simulink model "dsss"  (Simulink 7.1)
settings: Solver=ode45  StartTime=0.0  StopTime=0.80  RelTol=1e-3
libraries: simulink x264, dspbuff3 x24, dspxfrm3 x8, commsynccomp2 x5, dspsigops x4, dspobslib x4, dsparch4 x3, commutil2 x2, commseqgen2 x1, commfilt2 x1, commsink2 x1, dspspect3 x1
(part 1 of 4)
settings Model: Creator=Administrator  LastModifiedBy=Administrator

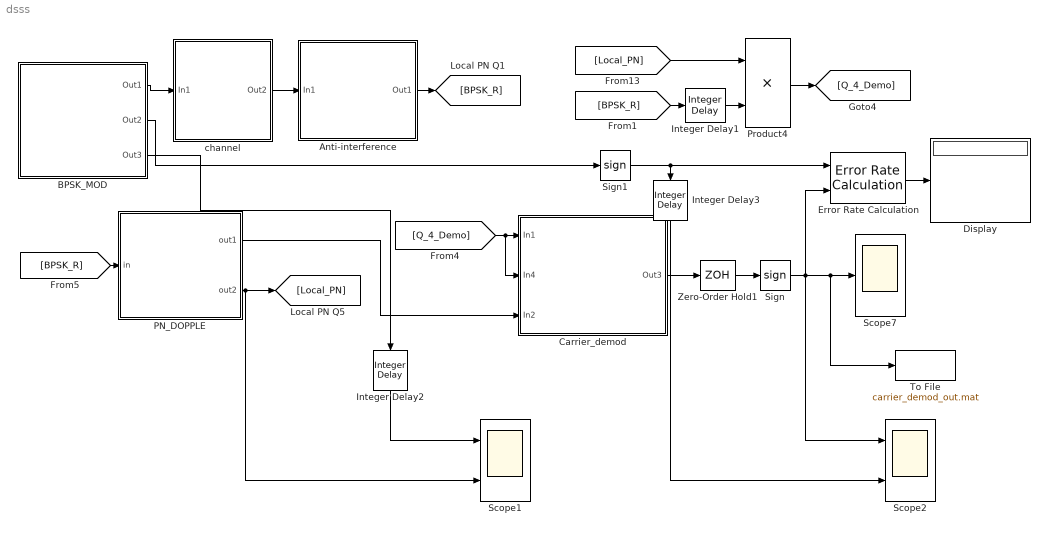
== system dsss ==
  Anti-interference : Subsystem
  BPSK_MOD : Subsystem
  Carrier_demod : Subsystem
  Display : Display
  Error Rate Calculation : commsink2/Error Rate Calculation  N=5  st_delay=0  cp_mode=Entire frame  subframe=[]  PMode=Port  WsName=ErrorVec  RsMode2=off  stop=off  numErr=100  maxBits=1e6
  Integer Delay1 : simulink/Discrete/Integer Delay  vinit=0.0  samptime=1/5.1e6  NumDelays=172
  Integer Delay2 : simulink/Discrete/Integer Delay  Orientation=down  vinit=0.0  samptime=1/5.1e6  NumDelays=22700
  Integer Delay3 : simulink/Discrete/Integer Delay  Orientation=down  vinit=0.0  samptime=1/1000  NumDelays=5
  PN_DOPPLE : Subsystem  TreatAsAtomicUnit=on
  Product4 : Product  OutDataType=sfix(16)  OutScaling=2^0  RndMeth=Zero
  Scope1 : Scope  NumInputPorts=2
      settings: YMin=-5~-5  YMax=5~5  SaveName=ScopeData3  MaxDataPoints=100000
  Scope2 : Scope  NumInputPorts=2
      settings: YMin=-5~-5  YMax=5~5  SaveName=ScopeData5  MaxDataPoints=100000
  Scope7 : Scope
      settings: SaveName=ScopeData7  MaxDataPoints=100000
  Sign : Signum
  Sign1 : Signum
  To File : ToFile  Filename=carrier_demod_out.mat
  Zero-Order Hold1 : ZeroOrderHold  SampleTime=1/1e3
  channel : Subsystem
  wires:
  BPSK_MOD/1(Out1) -> channel/1(In1)
  [BPSK_R] -> PN_DOPPLE/1(in)
  [Local_PN] -> Product4/1
  Product4/1 -> [Q_4_Demo]
  [BPSK_R] -> Integer Delay1/1
  Integer Delay1/1 -> Product4/2
  [Q_4_Demo] -> Carrier_demod/2(In4), Carrier_demod/1(In1)
  Carrier_demod/1(Out3) -> Zero-Order Hold1/1
  Zero-Order Hold1/1 -> Sign/1
  PN_DOPPLE/1(out1) -> Carrier_demod/3(In2)
  Sign/1 -> Error Rate Calculation/2, Scope2/1, Scope7/1, To File/1
  channel/1(Out2) -> Anti-interference/1(In1)
  Anti-interference/1(Out1) -> [BPSK_R]
  Error Rate Calculation/1 -> Display/1
  BPSK_MOD/2(Out2) -> Sign1/1
  PN_DOPPLE/2(out2) -> [Local_PN], Scope1/2
  BPSK_MOD/3(Out3) -> Integer Delay2/1
  Integer Delay2/1 -> Scope1/1
  Integer Delay3/1 -> Scope2/2
  Sign1/1 -> Error Rate Calculation/1, Integer Delay3/1

== system dsss/Anti-interference ==
  In1 : Inport  OutDataType=sfix(16)  OutScaling=2^0
  Add1 : Sum  Inputs=++++  OutDataType=sfix(16)  OutScaling=2^-10
  firstroad : Subsystem
  firstroad1 : Subsystem
  firstroad2 : Subsystem
  firstroad3 : Subsystem
  Out1 : Outport  OutDataType=sfix(16)  OutScaling=2^0
  wires:
  firstroad/1(Out1) -> Add1/1
  firstroad1/1(Out1) -> Add1/2
  firstroad2/1(Out1) -> Add1/3
  firstroad3/1(Out1) -> Add1/4
  In1/1 -> firstroad/1(In1), firstroad1/1(In1), firstroad2/1(In1), firstroad3/1(In1)
  Add1/1 -> Out1/1

== system dsss/BPSK_MOD ==
  Continuous-Time VCO1 : commsynccomp2/Continuous-Time VCO  SystemSampleTime=-1  Ac=1  Fc=510000  Kc=1000  Ph=pi/2
  PN_MOD : Subsystem
  Product6 : Product  OutDataType=sfix(16)  OutScaling=2^0  RndMeth=Zero
  Zero-Order Hold3 : ZeroOrderHold  SampleTime=1/5.1e6
  Out1 : Outport  OutDataType=sfix(16)  OutScaling=2^0
  Out2 : Outport  Port=2  OutDataType=sfix(16)  OutScaling=2^0
  Out3 : Outport  Port=3  OutDataType=sfix(16)  OutScaling=2^0
  wires:
  PN_MOD/1(Out1) -> Product6/2
  Continuous-Time VCO1/1 -> Zero-Order Hold3/1
  Zero-Order Hold3/1 -> Product6/1
  Product6/1 -> Out1/1
  PN_MOD/2(Out2) -> Out2/1
  PN_MOD/3(Out3) -> Out3/1

== system dsss/Carrier_demod ==
  note: 1.27e6 Hz
      |
      | 1/10.2e6
      |
      | 255K-300K
  In1 : Inport  OutDataType=sfix(16)  OutScaling=2^0
  In4 : Inport  Port=2  OutDataType=sfix(16)  OutScaling=2^0
  In2 : Inport  Port=3  OutDataType=sfix(16)  OutScaling=2^0
  Abs : Abs
  Add2 : Sum  Orientation=left  OutDataType=sfix(16)  OutScaling=2^-10
  Constant2 : Constant  OutDataType=sfix(16)  OutScaling=2^0
  Continuous-Time CO1 : commsynccomp2/Continuous-Time VCO  Orientation=left  SystemSampleTime=-1  Ac=2  Fc=5.1e5  Kc=1000  Ph=0
  Continuous-Time CO2 : commsynccomp2/Continuous-Time VCO  Orientation=left  SystemSampleTime=-1  Ac=2  Fc=5.1e5  Kc=1000  Ph=pi/2
  Digital Filter Design1 : dsparch4/Digital Filter Design  SystemSampleTime=-1  mwdsp_browser_bugfix_var=off
  Digital Filter Design2 : dsparch4/Digital Filter Design  SystemSampleTime=-1  mwdsp_browser_bugfix_var=off
  LF : Subsystem  Orientation=left
  Product : Product  OutDataType=sfix(16)  OutScaling=2^0  SaturateOnIntegerOverflow=on  OutDataTypeStr=Inherit: Same as first input
  Product2 : Product  Orientation=left  OutDataType=sfix(16)  OutScaling=2^0  SaturateOnIntegerOverflow=on  OutDataTypeStr=Inherit: Same as first input
  Product4 : Product  OutDataType=sfix(16)  OutScaling=2^0  SaturateOnIntegerOverflow=on  OutDataTypeStr=Inherit: Same as first input
  Scope{1..5} (5 alike) : Scope
      Scope1 settings: TimeRange=0.06427185951473757  YMin=-2  YMax=2  MaxDataPoints=100000
      Scope2 settings: TimeRange=0.06427185951473757  YMin=-2  YMax=2  SaveName=ScopeData6  MaxDataPoints=100000
      Scope3 settings: YMin=-2  YMax=2  SaveName=ScopeData35
      Scope4 settings: TimeRange=0.06427185951473757  YMin=-2  YMax=2  SaveName=ScopeData8  MaxDataPoints=100000
      Scope5 settings: TimeRange=0.06427185951473757  YMin=-2  YMax=2  SaveName=ScopeData2  MaxDataPoints=100000
  Subsystem2 : Subsystem  TreatAsAtomicUnit=on
  Switch2 : Switch  Criteria=u2 > Threshold
  Zero-Order Hold3 : ZeroOrderHold  Orientation=up  SampleTime=1/5.1e6
  Zero-Order Hold4 : ZeroOrderHold  SampleTime=1/1e5
  Zero-Order Hold5 : ZeroOrderHold  Orientation=down  SampleTime=1/5.1e6
  Zero-Order Hold6 : ZeroOrderHold  SampleTime=1/5.1e6
  Out3 : Outport  OutDataType=sfix(16)  OutScaling=2^0
  wires:
  Product2/1 -> LF/1(In2)
  Product/1 -> Digital Filter Design2/1
  Continuous-Time CO1/1 -> Zero-Order Hold3/1
  Digital Filter Design2/1 -> Product2/1, Abs/1, Zero-Order Hold6/1, Scope1/1  "unmoduled signal"
  In1/1 -> Product/1
  LF/1(Out1) -> Scope2/1, Add2/1
  Zero-Order Hold3/1 -> Product/2
  Subsystem2/1(Out1) -> Out3/1
  Constant2/1 -> Switch2/1
  Zero-Order Hold4/1 -> Switch2/2
  Switch2/1 -> Scope3/1, Subsystem2/Enable
  Abs/1 -> Zero-Order Hold4/1
  Zero-Order Hold6/1 -> Subsystem2/1(In1)
  Digital Filter Design1/1 -> Product2/2, Scope5/1
  Continuous-Time CO2/1 -> Zero-Order Hold5/1
  Product4/1 -> Digital Filter Design1/1
  In4/1 -> Product4/2
  Zero-Order Hold5/1 -> Product4/1
  Add2/1 -> Continuous-Time CO1/1, Continuous-Time CO2/1
  In2/1 -> Scope4/1, Add2/2

== system dsss/PN_DOPPLE ==
  in : Inport  OutDataType=sfix(16)  OutScaling=2^0
  "De-Carrier " : Subsystem
  FFT compensate : Subsystem
  Local PN : Subsystem
  MF Subsystem : Subsystem
  Magnitude FFT2 : dspspect3/Magnitude FFT  SystemSampleTime=-1  mag_or_magsq=Magnitude  fftLenInherit=off  fftsize=32
  MainTain System : Subsystem  TreatAsAtomicUnit=on
  Scope1 : Scope
      settings: TimeRange=0.06427185951473757  YMin=-2  YMax=2  SaveName=ScopeData14  MaxDataPoints=100000
  Scope3 : Scope
      settings: TimeRange=0.06427185951473757  YMin=-2  YMax=2  SaveName=ScopeData45  MaxDataPoints=100000
  Scope4 : Scope
      settings: TimeRange=0.06427185951473757  YMin=-2  YMax=2  SaveName=ScopeData21  MaxDataPoints=100000
  Sign : Signum
  Zero-Order Hold : ZeroOrderHold  SampleTime=1/255e3
  out1 : Outport  OutDataType=sfix(16)  OutScaling=2^0
  out2 : Outport  Port=2  OutDataType=sfix(16)  OutScaling=2^0
  wires:
  in/1 -> "De-Carrier "/1(in)
  FFT compensate/2(PN Peak) -> Scope3/1, Local PN/1(in)
  Zero-Order Hold/1 -> Sign/1, Scope4/1
  Sign/1 -> MF Subsystem/1(In1), Scope1/1, Local PN/2(in1)
  MF Subsystem/1(bus Out1) -> Magnitude FFT2/1
  Magnitude FFT2/1 -> FFT compensate/1(In1)
  FFT compensate/1(FFT compensate positive) -> MainTain System/1(In1), MainTain System/Trigger
  MainTain System/1(Out1) -> out1/1
  "De-Carrier "/1(out) -> Zero-Order Hold/1
  Local PN/1(1 0 0 1 1 1 0 1) -> out2/1

== system dsss/channel ==
  In1 : Inport  OutDataType=sfix(16)  OutScaling=2^0
  AWGN Channel : commchan3/AWGN Channel  SystemSampleTime=-1  seed=67  noiseMode="Signal to noise ratio  (SNR)"  EbNodB=10  EsNodB=10  SNRdB=-3.95  bitsPerSym=1  Ps=1  Tsym=1  variance=1
  Add : Sum  OutDataType=sfix(16)  OutScaling=2^-10
  Scope9 : Scope
      settings: TimeRange=0.06427185951473757  YMin=0  YMax=14
  Zero-Order Hold1 : ZeroOrderHold  SampleTime=1/5.1e6
  Zero-Order Hold3 : ZeroOrderHold  SampleTime=1/5.1e6
  zhaidaigr : Subsystem
  Out2 : Outport  OutDataType=sfix(16)  OutScaling=2^0
  wires:
  Zero-Order Hold3/1 -> Scope9/1, AWGN Channel/1
  In1/1 -> Zero-Order Hold3/1
  zhaidaigr/1(Out1) -> Add/2
  Add/1 -> Out2/1
  Zero-Order Hold1/1 -> Add/1
  AWGN Channel/1 -> Zero-Order Hold1/1

== system dsss/Anti-interference/firstroad ==
  In1 : Inport  OutDataType=sfix(16)  OutScaling=2^0
  Complex to Magnitude-Angle : ComplexToMagnitudeAngle
  all : Subsystem
  inteference_delieve : Subsystem
  inverse_convertion : Subsystem  Orientation=left
  threshold : Subsystem
  Out1 : Outport  Orientation=left  OutDataType=sfix(16)  OutScaling=2^0
  wires:
  all/1(Out1) -> Complex to Magnitude-Angle/1
  Complex to Magnitude-Angle/1 -> threshold/1(In1), inteference_delieve/1(In1)
  Complex to Magnitude-Angle/2 -> inverse_convertion/1(In1)
  inteference_delieve/1(Out1) -> inverse_convertion/2(In2)
  threshold/1(Out1) -> inteference_delieve/2(In2)
  In1/1 -> all/1(In1)
  inverse_convertion/1(Out1) -> Out1/1

== system dsss/Anti-interference/firstroad1 ==
  In1 : Inport  OutDataType=sfix(16)  OutScaling=2^0
  Complex to Magnitude-Angle : ComplexToMagnitudeAngle
  all : Subsystem
  inteference_delieve : Subsystem
  inverse_convertion : Subsystem  Orientation=left
  threshold : Subsystem
  Out1 : Outport  Orientation=left  OutDataType=sfix(16)  OutScaling=2^0
  wires:
  inverse_convertion/1(Out1) -> Out1/1
  In1/1 -> all/1(In1)
  threshold/1(Out1) -> inteference_delieve/2(In2)
  inteference_delieve/1(Out1) -> inverse_convertion/2(In2)
  Complex to Magnitude-Angle/2 -> inverse_convertion/1(In1)
  Complex to Magnitude-Angle/1 -> inteference_delieve/1(In1), threshold/1(In1)
  all/1(Out1) -> Complex to Magnitude-Angle/1

== system dsss/Anti-interference/firstroad2 ==
  In1 : Inport  OutDataType=sfix(16)  OutScaling=2^0
  Complex to Magnitude-Angle : ComplexToMagnitudeAngle
  all : Subsystem
  inteference_delieve : Subsystem
  inverse_convertion : Subsystem  Orientation=left
  threshold : Subsystem
  Out1 : Outport  Orientation=left  OutDataType=sfix(16)  OutScaling=2^0
  wires:
  all/1(Out1) -> Complex to Magnitude-Angle/1
  Complex to Magnitude-Angle/1 -> threshold/1(In1), inteference_delieve/1(In1)
  Complex to Magnitude-Angle/2 -> inverse_convertion/1(In1)
  inteference_delieve/1(Out1) -> inverse_convertion/2(In2)
  threshold/1(Out1) -> inteference_delieve/2(In2)
  In1/1 -> all/1(In1)
  inverse_convertion/1(Out1) -> Out1/1

== system dsss/Anti-interference/firstroad3 ==
  In1 : Inport  OutDataType=sfix(16)  OutScaling=2^0
  Complex to Magnitude-Angle : ComplexToMagnitudeAngle
  all : Subsystem
  inteference_delieve : Subsystem
  inverse_convertion : Subsystem  Orientation=left
  threshold : Subsystem
  Out1 : Outport  Orientation=left  OutDataType=sfix(16)  OutScaling=2^0
  wires:
  inverse_convertion/1(Out1) -> Out1/1
  In1/1 -> all/1(In1)
  threshold/1(Out1) -> inteference_delieve/2(In2)
  inteference_delieve/1(Out1) -> inverse_convertion/2(In2)
  Complex to Magnitude-Angle/2 -> inverse_convertion/1(In1)
  Complex to Magnitude-Angle/1 -> inteference_delieve/1(In1), threshold/1(In1)
  all/1(Out1) -> Complex to Magnitude-Angle/1

== system dsss/BPSK_MOD/PN_MOD ==
  1 0 0 0 1 1 1 0 2 : commseqgen2/PN Sequence Generator  poly=[1 0 0 0 1 1 1 0 1]  ini_sta=[0 0 0 0 0 0 0 1]  outBitMaskSource=Dialog parameter  shift=0  Ts=1/2.55e5  frameBased=off  sampPerFrame=1  reset=off  bitPackedOutputs=off  outDataType=double  numPackedBits=8  bitPackDataSigned=off  bitPackedOutDType=double
  From File : FromFile  FileName=encode_out.mat  SampleTime=1/1000
  Product5 : Product  OutDataType=sfix(16)  OutScaling=2^0  RndMeth=Zero
  Unipolar to Bipolar Converter : commutil2/Unipolar to Bipolar Converter  SystemSampleTime=-1  M=2  polarity=Positive  dataType=Same as input
  Out1 : Outport
  Out2 : Outport  Port=2
  Out3 : Outport  Port=3
  wires:
  1 0 0 0 1 1 1 0 2/1 -> Unipolar to Bipolar Converter/1
  Unipolar to Bipolar Converter/1 -> Product5/1, Out3/1
  From File/1 -> Product5/2, Out2/1
  Product5/1 -> Out1/1

== system dsss/Carrier_demod/LF ==
  In2 : Inport  OutDataType=sfix(16)  OutScaling=2^0
  Gain : Gain  Gain=0.4  ParameterDataType=sfix(16)  ParameterScaling=2^0  OutDataType=sfix(16)  OutScaling=2^0  SaturateOnIntegerOverflow=on  OutDataTypeStr=Inherit: Same as input  ParamDataTypeStr=Inherit: Same as input
  Gain1 : Gain  Gain=0.02  ParameterDataType=sfix(16)  ParameterScaling=2^0  OutDataType=sfix(16)  OutScaling=2^0  SaturateOnIntegerOverflow=on  OutDataTypeStr=Inherit: Same as input  ParamDataTypeStr=Inherit: Same as input
  Sum1 : Sum  Inputs=|++  OutDataType=sfix(16)  OutScaling=2^0  SaturateOnIntegerOverflow=on  InputSameDT=on  OutDataTypeStr=Inherit: Same as first input
  Sum2 : Sum  Inputs=|++  OutDataType=sfix(16)  OutScaling=2^0  SaturateOnIntegerOverflow=on  InputSameDT=on  OutDataTypeStr=Inherit: Same as first input
  Unit Delay : UnitDelay  Orientation=left  SampleTime=1/1e5
  Out1 : Outport  OutDataType=sfix(16)  OutScaling=2^0
  wires:
  In2/1 -> Gain1/1, Gain/1
  Gain1/1 -> Sum2/1
  Unit Delay/1 -> Sum2/2
  Gain/1 -> Sum1/1
  Sum1/1 -> Out1/1
  Sum2/1 -> Sum1/2, Unit Delay/1

== system dsss/Carrier_demod/Subsystem2 ==
  In1 : Inport  OutDataType=sfix(16)  OutScaling=2^0
  Enable : EnablePort
  Gain : Gain  Gain=1/100  ParameterDataType=sfix(16)  ParameterScaling=2^0  OutDataType=sfix(16)  OutScaling=2^0
  Integrate and Dump : commfilt2/Integrate and Dump  DialogController=commDDGCreate  DialogControllerArgs=DataTag18  obssamples=100  offsetsamples=0  nodump=off  roundingMode=Floor  overflowMode=off
  Out1 : Outport  OutDataType=sfix(16)  OutScaling=2^0
  wires:
  Integrate and Dump/1 -> Gain/1
  In1/1 -> Integrate and Dump/1
  Gain/1 -> Out1/1

== system dsss/PN_DOPPLE/De-Carrier  ==
  note: 5.1e5 Hz
      |
      | 1/5.1e6
      |
      | 255K-300K
  in : Inport  OutDataType=sfix(16)  OutScaling=2^0
  Continuous-Time VCO1 : commsynccomp2/Continuous-Time VCO  SystemSampleTime=-1  Ac=1  Fc=5.1e5  Kc=1000  Ph=pi/2
  Digital Filter Design4 : dsparch4/Digital Filter Design  SystemSampleTime=-1  mwdsp_browser_bugfix_var=off
  Product1 : Product  OutDataType=sfix(16)  OutScaling=2^0  RndMeth=Zero
  Scope1 : Scope
      settings: SaveName=ScopeData4  MaxDataPoints=100000
  Scope3 : Scope
      settings: SaveName=ScopeData16  MaxDataPoints=100000
  Zero-Order Hold2 : ZeroOrderHold  SampleTime=1/5.1e6
  out : Outport  OutDataType=sfix(16)  OutScaling=2^0
  wires:
  in/1 -> Product1/2
  Product1/1 -> Scope3/1, Digital Filter Design4/1
  Digital Filter Design4/1 -> out/1, Scope1/1
  Continuous-Time VCO1/1 -> Zero-Order Hold2/1
  Zero-Order Hold2/1 -> Product1/1

== system dsss/PN_DOPPLE/FFT compensate ==
  In1 : Inport  OutDataType=sfix(16)  OutScaling=2^0
  Demux : Demux  Outputs=32
  Product1 : Product  OutDataType=sfix(16)  OutScaling=2^0  RndMeth=Zero
  Product8 : Product  OutDataType=sfix(16)  OutScaling=2^0  RndMeth=Zero
  Rate Transition1 : RateTransition  Deterministic=off  OutPortSampleTime=1/5.1e6
  Rate Transition2 : RateTransition  Deterministic=off  OutPortSampleTime=1/5.1e6
  Rate Transition3 : RateTransition  Deterministic=off  OutPortSampleTime=1/5.1e6
  Scope{1..2,4..7} (6 alike) : Scope  NumInputPorts=3
      Scope1 settings: TimeRange=0.06427185951473757  YMin=0~-5~-5  YMax=14~5~5  SaveName=ScopeData9  MaxDataPoints=100000
      Scope2 settings: TimeRange=0.06427185951473757  YMin=0~-5~-5  YMax=14~5~5  SaveName=ScopeData11  MaxDataPoints=100000
      Scope4 settings: TimeRange=0.06427185951473757  YMin=0~-5~-5  YMax=14~5~5  SaveName=ScopeData12  MaxDataPoints=100000
      Scope5 settings: TimeRange=0.06427185951473757  YMin=0~-5~-5  YMax=14~5~5  SaveName=ScopeData13  MaxDataPoints=100000
      Scope6 settings: TimeRange=0.06427185951473757  YMin=0~-5~-5  YMax=14~5~5  SaveName=ScopeData33  MaxDataPoints=100000
      Scope7 settings: TimeRange=0.06427185951473757  YMin=0~-5~-5  YMax=14~5~5  SaveName=ScopeData47  MaxDataPoints=100000
  Scope14 : Scope
      settings: SaveName=ScopeData24  MaxDataPoints=100000
  Scope3 : Scope
      settings: SaveName=ScopeData27  MaxDataPoints=100000
  Step : Step  Time=0.001  SampleTime=0
  Step1 : Step  Time=0.001  SampleTime=0
  Subsystem : Subsystem
  FFT compensate positive : Outport  OutDataType=sfix(16)  OutScaling=2^0
  PN Peak : Outport  Port=2  OutDataType=sfix(16)  OutScaling=2^0
  wires:
  Demux/3 -> Subsystem/3(In3), Scope2/3
  Demux/2 -> Subsystem/2(In2), Scope2/2
  Demux/4 -> Scope1/1, Subsystem/4(In4)
  Demux/5 -> Scope1/2, Subsystem/5(In5)
  Demux/6 -> Scope1/3, Subsystem/6(In6)
  Demux/7 -> Subsystem/7(In7), Scope4/1
  Demux/8 -> Subsystem/8(In8), Scope4/2
  Demux/9 -> Subsystem/9(In9), Scope4/3
  Demux/10 -> Subsystem/10(In10), Scope5/1
  Demux/11 -> Subsystem/11(In11), Scope5/2
  Demux/12 -> Subsystem/12(In12), Scope5/3
  Demux/13 -> Subsystem/13(In13), Scope6/1
  Demux/14 -> Subsystem/14(In14), Scope6/2
  Demux/15 -> Subsystem/15(In15), Scope6/3
  In1/1 -> Demux/1
  Demux/1 -> Subsystem/1(In1), Scope2/1
  Subsystem/1(Out1) -> Scope14/1, Product1/1
  Step/1 -> Rate Transition3/1
  Product8/1 -> Rate Transition1/1
  Subsystem/2(Out2) -> Rate Transition2/1
  Rate Transition1/1 -> PN Peak/1, Scope3/1
  Rate Transition2/1 -> Product8/1
  Demux/16 -> Subsystem/16(In16), Scope7/1
  Demux/17 -> Scope7/2
  Demux/18 -> Scope7/3
  Rate Transition3/1 -> Product8/2
  Step1/1 -> Product1/2
  Product1/1 -> FFT compensate positive/1

== system dsss/PN_DOPPLE/Local PN ==
  in : Inport  OutDataType=sfix(16)  OutScaling=2^0
  in1 : Inport  Port=2  OutDataType=sfix(16)  OutScaling=2^0
  Scope{1..3,5} (4 alike) : Scope
      Scope1 settings: TimeRange=0.06427185951473757  YMin=-2  YMax=2  SaveName=ScopeData23  MaxDataPoints=100000
      Scope2 settings: TimeRange=0.06427185951473757  YMin=-2  YMax=2  SaveName=ScopeData29  MaxDataPoints=100000
      Scope3 settings: TimeRange=0.06427185951473757  YMin=-2  YMax=2  SaveName=ScopeData18  MaxDataPoints=100000
      Scope5 settings: TimeRange=0.06427185951473757  YMin=-2  YMax=2  SaveName=ScopeData30  MaxDataPoints=100000
  local PN sequence Include Track : Subsystem  TreatAsAtomicUnit=on
  logic control : Subsystem  TreatAsAtomicUnit=on
  threshold deside : Subsystem  TreatAsAtomicUnit=on
  threshold deside stop and start : Subsystem
  1 0 0 1 1 1 0 1 : Outport  OutDataType=sfix(16)  OutScaling=2^0
  wires:
  logic control/1(Out2) -> Scope5/1, local PN sequence Include Track/Enable
  threshold deside/1(Out2) -> logic control/1(In1), threshold deside stop and start/1(In1)
  threshold deside stop and start/1(Out1) -> threshold deside/Enable, Scope3/1
  [A] -> threshold deside stop and start/2(In2)
  in/1 -> threshold deside/1(In1), Scope2/1
  local PN sequence Include Track/1("1 0 0 1 1 1 0 1 ") -> 1 0 0 1 1 1 0 1/1, Scope1/1
  ? -> local PN sequence Include Track/1(B)

== system dsss/PN_DOPPLE/MF Subsystem ==
  In1 : Inport  OutDataType=sfix(16)  OutScaling=2^0
  Add : Sum  Inputs=++++++++++++++++++++++++++++++++  OutDataType=sfix(16)  OutScaling=2^-10
  MF array : Subsystem
  Mux : Mux  Inputs=32
  Scope14 : Scope
      settings: SaveName=ScopeData34  MaxDataPoints=100000
  Zero-Order Hold : ZeroOrderHold  SampleTime=1/255000
  bus Out1 : Outport  OutDataType=sfix(16)  OutScaling=2^0
  wires:
  In1/1 -> Zero-Order Hold/1
  Zero-Order Hold/1 -> MF array/1(In1)
  Mux/1 -> bus Out1/1
  Add/1 -> Scope14/1
  MF array/1(Out1) -> Mux/1, Add/1
  MF array/2(Out2) -> Mux/2, Add/2
  MF array/3(Out3) -> Mux/3, Add/3
  MF array/4(Out4) -> Mux/4, Add/4
  MF array/5(Out5) -> Mux/5, Add/5
  MF array/6(Out6) -> Mux/6, Add/6
  MF array/7(Out7) -> Mux/7, Add/7
  MF array/8(Out8) -> Mux/8, Add/8
  MF array/9(Out9) -> Mux/9, Add/9
  MF array/10(Out10) -> Mux/10, Add/10
  MF array/11(Out11) -> Mux/11, Add/11
  MF array/12(Out12) -> Mux/12, Add/12
  MF array/13(Out13) -> Mux/13, Add/13
  MF array/14(Out14) -> Mux/14, Add/14
  MF array/15(Out15) -> Mux/15, Add/15
  MF array/16(Out16) -> Mux/16, Add/16
  MF array/17(Out17) -> Mux/17, Add/17
  MF array/18(Out18) -> Mux/18, Add/18
  MF array/19(Out19) -> Mux/19, Add/19
  MF array/20(Out20) -> Mux/20, Add/20
  MF array/21(Out21) -> Mux/21, Add/21
  MF array/22(Out22) -> Mux/22, Add/22
  MF array/23(Out23) -> Mux/23, Add/23
  MF array/24(Out24) -> Mux/24, Add/24
  MF array/25(Out25) -> Mux/25, Add/25
  MF array/26(Out26) -> Mux/26, Add/26
  MF array/27(Out27) -> Mux/27, Add/27
  MF array/28(Out28) -> Mux/28, Add/28
  MF array/29(Out29) -> Mux/29, Add/29
  MF array/30(Out30) -> Mux/30, Add/30
  MF array/31(Out31) -> Mux/31, Add/31
  MF array/32(Out32) -> Mux/32, Add/32

== system dsss/PN_DOPPLE/MainTain System ==
  In1 : Inport  OutDataType=sfix(16)  OutScaling=2^0
  Trigger : TriggerPort
  Out1 : Outport  OutDataType=sfix(16)  OutScaling=2^0
  wires:
  In1/1 -> Out1/1

== system dsss/channel/zhaidaigr ==
  Sine Wave : Sin  Amplitude=30  Frequency=10.2e5*pi  SampleTime=0
  Zero-Order Hold1 : ZeroOrderHold  SampleTime=1/5.1e6
  Out1 : Outport  OutDataType=sfix(16)  OutScaling=2^0
  wires:
  Zero-Order Hold1/1 -> Out1/1
  Sine Wave/1 -> Zero-Order Hold1/1

== system dsss/Anti-interference/firstroad/all ==
  In1 : Inport  OutDataType=sfix(16)  OutScaling=2^0
  Buffer1 : dspbuff3/Buffer  N=8192  V=0  ic=0
  FFT1 : dspxfrm3/FFT  DialogController=dspDDGCreate  DialogControllerArgs=DataTag0  CompMethod=Table lookup  TableOpt=HYBRID  TableOptActive=Speed  BitRevOrder=off  InheritFFTLength=on  FFTLength=64  SkipNorm=off  roundingMode=Floor  overflowMode=off
  Window Function : dspsigops/Window Function  DialogController=dspDDGCreate  DialogControllerArgs=DataTag1  winmode=Apply window to input  wintype=Chebyshev  sampmode=Continuous  samptime=1  N=64  Rs=80  beta=10  winsamp=Symmetric  UserWindow=hamming  OptParams=off  UserParams={'symmetric'}  dataType=double  isSigned=on  wordLen=16  udDataType=sfix(16)  fracBitsMode=Best precision  numFracBits=15  roundingMode=Floor  overflowMode=off  numSidelobes=4  sidelobeLevel=-30
  Out1 : Outport  OutDataType=sfix(16)  OutScaling=2^0
  wires:
  Buffer1/1 -> Window Function/1
  FFT1/1 -> Out1/1
  In1/1 -> Buffer1/1
  Window Function/1 -> FFT1/1

== system dsss/Anti-interference/firstroad/inteference_delieve ==
  In1 : Inport  OutDataType=sfix(16)  OutScaling=2^0
  In2 : Inport  Port=2  OutDataType=sfix(16)  OutScaling=2^0
  Buffer1 : dspbuff3/Buffer  N=8192  V=0  ic=0
  Frame Conversion : FrameConversion
  Frame Conversion1 : FrameConversion  Orientation=left  OutFrame=Sample-based
  Gain : Gain  Gain=0.1  ParameterDataType=sfix(16)  ParameterScaling=2^0  OutDataType=sfix(16)  OutScaling=2^0
  Subtract : Sum  Inputs=+-  OutDataType=sfix(16)  OutScaling=2^-10
  Switch : Switch
  Unbuffer : dspbuff3/Unbuffer  ic=0
  Out1 : Outport  Orientation=left  OutDataType=sfix(16)  OutScaling=2^0
  wires:
  Unbuffer/1 -> Subtract/1, Switch/3
  Frame Conversion/1 -> Unbuffer/1
  In2/1 -> Subtract/2, Gain/1
  Subtract/1 -> Switch/2
  Gain/1 -> Switch/1
  Switch/1 -> Buffer1/1
  Buffer1/1 -> Frame Conversion1/1
  In1/1 -> Frame Conversion/1
  Frame Conversion1/1 -> Out1/1

== system dsss/Anti-interference/firstroad/inverse_convertion ==
  In1 : Inport  Orientation=left  OutDataType=sfix(16)  OutScaling=2^0
  In2 : Inport  Orientation=left  Port=2  OutDataType=sfix(16)  OutScaling=2^0
  Buffer2 : dspbuff3/Buffer  Orientation=left  N=8192  V=0  ic=0
  Complex to Real-Imag : ComplexToRealImag  Orientation=left  Output=Real
  Frame Conversion2 : FrameConversion  Orientation=left
  Frame Conversion3 : FrameConversion  Orientation=left  OutFrame=Sample-based
  IFFT : dspxfrm3/IFFT  Orientation=left  DialogController=dspDDGCreate  DialogControllerArgs=DataTag2  CompMethod=Table lookup  TableOpt=HYBRID  TableOptActive=Speed  BitRevOrder=off  cs_in=off  SkipNorm=on  InheritFFTLength=on  FFTLength=64  mode=Complex  outSamplingMode=Frame based  roundingMode=Floor  overflowMode=off
  Integer Delay : simulink/Discrete/Integer Delay  Orientation=left  vinit=0.0  samptime=-1  NumDelays=6144
  Magnitude-Angle to Complex : MagnitudeAngleToComplex  Orientation=left
  Unbuffer1 : dspbuff3/Unbuffer  Orientation=left  ic=0
  Unbuffer2 : dspbuff3/Unbuffer  Orientation=left  ic=0
  Out1 : Outport  Orientation=left  OutDataType=sfix(16)  OutScaling=2^0
  wires:
  Frame Conversion2/1 -> Unbuffer1/1
  Unbuffer1/1 -> Buffer2/1
  Buffer2/1 -> Frame Conversion3/1
  Magnitude-Angle to Complex/1 -> IFFT/1
  IFFT/1 -> Integer Delay/1
  Unbuffer2/1 -> Complex to Real-Imag/1
  Frame Conversion3/1 -> Magnitude-Angle to Complex/2
  Complex to Real-Imag/1 -> Out1/1
  In1/1 -> Frame Conversion2/1
  In2/1 -> Magnitude-Angle to Complex/1
  Integer Delay/1 -> Unbuffer2/1

== system dsss/Anti-interference/firstroad/threshold ==
  In1 : Inport  OutDataType=sfix(16)  OutScaling=2^0
  Add1 : Sum  OutDataType=sfix(16)  OutScaling=2^-10
  Constant : Constant  Value=8192  OutDataType=sfix(16)  OutScaling=2^0
  Constant1 : Constant  Value=400  OutDataType=sfix(16)  OutScaling=2^0
  Display6 : Display
  Divide : Product  Inputs=*/  OutDataType=sfix(16)  OutScaling=2^-10
  Gain : Gain  Gain=0.3  ParameterDataType=sfix(16)  ParameterScaling=2^0  OutDataType=sfix(16)  OutScaling=2^0
  Matrix Sum : dspobslib/Matrix Sum  DialogController=dspDDGCreate  DialogControllerArgs=DataTag3  Dim=Columns  roundingMode=Floor  overflowMode=off
  Rate Transition1 : RateTransition  Deterministic=off  OutPortSampleTime=8192/5.1e6
  Rate Transition2 : RateTransition  Orientation=down  Deterministic=off  OutPortSampleTime=1/5.1e6
  Zero-Order Hold5 : ZeroOrderHold  SampleTime=1/5.1e6
  Out1 : Outport  OutDataType=sfix(16)  OutScaling=2^0
  wires:
  Matrix Sum/1 -> Divide/1
  Divide/1 -> Gain/1
  Gain/1 -> Rate Transition2/1
  Add1/1 -> Display6/1, Out1/1
  In1/1 -> Matrix Sum/1
  Constant1/1 -> Zero-Order Hold5/1
  Rate Transition1/1 -> Divide/2
  Constant/1 -> Rate Transition1/1
  Zero-Order Hold5/1 -> Add1/2
  Rate Transition2/1 -> Add1/1

== system dsss/Anti-interference/firstroad1/all ==
  In1 : Inport  OutDataType=sfix(16)  OutScaling=2^0
  Buffer1 : dspbuff3/Buffer  N=8192  V=0  ic=0
  FFT1 : dspxfrm3/FFT  DialogController=dspDDGCreate  DialogControllerArgs=DataTag4  CompMethod=Table lookup  TableOpt=HYBRID  TableOptActive=Speed  BitRevOrder=off  InheritFFTLength=on  FFTLength=64  SkipNorm=off  roundingMode=Floor  overflowMode=off
  Integer Delay : simulink/Discrete/Integer Delay  vinit=0.0  samptime=-1  NumDelays=2048
  Window Function : dspsigops/Window Function  DialogController=dspDDGCreate  DialogControllerArgs=DataTag5  winmode=Apply window to input  wintype=Chebyshev  sampmode=Continuous  samptime=1  N=64  Rs=80  beta=10  winsamp=Symmetric  UserWindow=hamming  OptParams=off  UserParams={'symmetric'}  dataType=double  isSigned=on  wordLen=16  udDataType=sfix(16)  fracBitsMode=Best precision  numFracBits=15  roundingMode=Floor  overflowMode=off  numSidelobes=4  sidelobeLevel=-30
  Out1 : Outport  OutDataType=sfix(16)  OutScaling=2^0
  wires:
  Window Function/1 -> FFT1/1
  In1/1 -> Buffer1/1
  FFT1/1 -> Out1/1
  Buffer1/1 -> Integer Delay/1
  Integer Delay/1 -> Window Function/1

== system dsss/Anti-interference/firstroad1/inteference_delieve ==
  In1 : Inport  OutDataType=sfix(16)  OutScaling=2^0
  In2 : Inport  Port=2  OutDataType=sfix(16)  OutScaling=2^0
  Buffer1 : dspbuff3/Buffer  N=8192  V=0  ic=0
  Frame Conversion : FrameConversion
  Frame Conversion1 : FrameConversion  Orientation=left  OutFrame=Sample-based
  Gain : Gain  Gain=0.1  ParameterDataType=sfix(16)  ParameterScaling=2^0  OutDataType=sfix(16)  OutScaling=2^0
  Subtract : Sum  Inputs=+-  OutDataType=sfix(16)  OutScaling=2^-10
  Switch : Switch
  Unbuffer : dspbuff3/Unbuffer  ic=0
  Out1 : Outport  Orientation=left  OutDataType=sfix(16)  OutScaling=2^0
  wires:
  Frame Conversion1/1 -> Out1/1
  In1/1 -> Frame Conversion/1
  Buffer1/1 -> Frame Conversion1/1
  Switch/1 -> Buffer1/1
  Gain/1 -> Switch/1
  Subtract/1 -> Switch/2
  In2/1 -> Gain/1, Subtract/2
  Frame Conversion/1 -> Unbuffer/1
  Unbuffer/1 -> Switch/3, Subtract/1

== system dsss/Anti-interference/firstroad1/inverse_convertion ==
  In1 : Inport  Orientation=left  OutDataType=sfix(16)  OutScaling=2^0
  In2 : Inport  Orientation=left  Port=2  OutDataType=sfix(16)  OutScaling=2^0
  Buffer2 : dspbuff3/Buffer  Orientation=left  N=8192  V=0  ic=0
  Complex to Real-Imag : ComplexToRealImag  Orientation=left  Output=Real
  Frame Conversion2 : FrameConversion  Orientation=left
  Frame Conversion3 : FrameConversion  Orientation=left  OutFrame=Sample-based
  IFFT : dspxfrm3/IFFT  Orientation=left  DialogController=dspDDGCreate  DialogControllerArgs=DataTag6  CompMethod=Table lookup  TableOpt=HYBRID  TableOptActive=Speed  BitRevOrder=off  cs_in=off  SkipNorm=on  InheritFFTLength=on  FFTLength=64  mode=Complex  outSamplingMode=Frame based  roundingMode=Floor  overflowMode=off
  Integer Delay : simulink/Discrete/Integer Delay  Orientation=left  vinit=0.0  samptime=-1  NumDelays=4096
  Magnitude-Angle to Complex : MagnitudeAngleToComplex  Orientation=left
  Unbuffer1 : dspbuff3/Unbuffer  Orientation=left  ic=0
  Unbuffer2 : dspbuff3/Unbuffer  Orientation=left  ic=0
  Out1 : Outport  Orientation=left  OutDataType=sfix(16)  OutScaling=2^0
  wires:
  Integer Delay/1 -> Unbuffer2/1
  In2/1 -> Magnitude-Angle to Complex/1
  In1/1 -> Frame Conversion2/1
  Complex to Real-Imag/1 -> Out1/1
  Frame Conversion3/1 -> Magnitude-Angle to Complex/2
  Unbuffer2/1 -> Complex to Real-Imag/1
  IFFT/1 -> Integer Delay/1
  Magnitude-Angle to Complex/1 -> IFFT/1
  Buffer2/1 -> Frame Conversion3/1
  Unbuffer1/1 -> Buffer2/1
  Frame Conversion2/1 -> Unbuffer1/1

== system dsss/Anti-interference/firstroad1/threshold ==
  In1 : Inport  OutDataType=sfix(16)  OutScaling=2^0
  Add1 : Sum  OutDataType=sfix(16)  OutScaling=2^-10
  Constant : Constant  Value=8192  OutDataType=sfix(16)  OutScaling=2^0
  Constant1 : Constant  Value=400  OutDataType=sfix(16)  OutScaling=2^0
  Display6 : Display
  Divide : Product  Inputs=*/  OutDataType=sfix(16)  OutScaling=2^-10
  Gain : Gain  Gain=0.3  ParameterDataType=sfix(16)  ParameterScaling=2^0  OutDataType=sfix(16)  OutScaling=2^0
  Matrix Sum : dspobslib/Matrix Sum  DialogController=dspDDGCreate  DialogControllerArgs=DataTag7  Dim=Columns  roundingMode=Floor  overflowMode=off
  Rate Transition1 : RateTransition  Deterministic=off  OutPortSampleTime=8192/5.1e6
  Rate Transition2 : RateTransition  Orientation=down  Deterministic=off  OutPortSampleTime=1/5.1e6
  Zero-Order Hold5 : ZeroOrderHold  SampleTime=1/5.1e6
  Out1 : Outport  OutDataType=sfix(16)  OutScaling=2^0
  wires:
  Rate Transition2/1 -> Add1/1
  Zero-Order Hold5/1 -> Add1/2
  Constant/1 -> Rate Transition1/1
  Rate Transition1/1 -> Divide/2
  Constant1/1 -> Zero-Order Hold5/1
  In1/1 -> Matrix Sum/1
  Add1/1 -> Out1/1, Display6/1
  Gain/1 -> Rate Transition2/1
  Divide/1 -> Gain/1
  Matrix Sum/1 -> Divide/1

== system dsss/Anti-interference/firstroad2/all ==
  In1 : Inport  OutDataType=sfix(16)  OutScaling=2^0
  Buffer1 : dspbuff3/Buffer  N=8192  V=0  ic=0
  FFT1 : dspxfrm3/FFT  DialogController=dspDDGCreate  DialogControllerArgs=DataTag8  CompMethod=Table lookup  TableOpt=HYBRID  TableOptActive=Speed  BitRevOrder=off  InheritFFTLength=on  FFTLength=64  SkipNorm=off  roundingMode=Floor  overflowMode=off
  Integer Delay : simulink/Discrete/Integer Delay  vinit=0.0  samptime=-1  NumDelays=4096
  Window Function : dspsigops/Window Function  DialogController=dspDDGCreate  DialogControllerArgs=DataTag9  winmode=Apply window to input  wintype=Chebyshev  sampmode=Continuous  samptime=1  N=64  Rs=80  beta=10  winsamp=Symmetric  UserWindow=hamming  OptParams=off  UserParams={'symmetric'}  dataType=double  isSigned=on  wordLen=16  udDataType=sfix(16)  fracBitsMode=Best precision  numFracBits=15  roundingMode=Floor  overflowMode=off  numSidelobes=4  sidelobeLevel=-30
  Out1 : Outport  OutDataType=sfix(16)  OutScaling=2^0
  wires:
  Integer Delay/1 -> Window Function/1
  Buffer1/1 -> Integer Delay/1
  FFT1/1 -> Out1/1
  In1/1 -> Buffer1/1
  Window Function/1 -> FFT1/1

== system dsss/Anti-interference/firstroad2/inteference_delieve ==
  In1 : Inport  OutDataType=sfix(16)  OutScaling=2^0
  In2 : Inport  Port=2  OutDataType=sfix(16)  OutScaling=2^0
  Buffer1 : dspbuff3/Buffer  N=8192  V=0  ic=0
  Frame Conversion : FrameConversion
  Frame Conversion1 : FrameConversion  Orientation=left  OutFrame=Sample-based
  Gain : Gain  Gain=0.1  ParameterDataType=sfix(16)  ParameterScaling=2^0  OutDataType=sfix(16)  OutScaling=2^0
  Subtract : Sum  Inputs=+-  OutDataType=sfix(16)  OutScaling=2^-10
  Switch : Switch
  Unbuffer : dspbuff3/Unbuffer  ic=0
  Out1 : Outport  Orientation=left  OutDataType=sfix(16)  OutScaling=2^0
  wires:
  Unbuffer/1 -> Subtract/1, Switch/3
  Frame Conversion/1 -> Unbuffer/1
  In2/1 -> Subtract/2, Gain/1
  Subtract/1 -> Switch/2
  Gain/1 -> Switch/1
  Switch/1 -> Buffer1/1
  Buffer1/1 -> Frame Conversion1/1
  In1/1 -> Frame Conversion/1
  Frame Conversion1/1 -> Out1/1

== system dsss/Anti-interference/firstroad2/inverse_convertion ==
  In1 : Inport  Orientation=left  OutDataType=sfix(16)  OutScaling=2^0
  In2 : Inport  Orientation=left  Port=2  OutDataType=sfix(16)  OutScaling=2^0
  Buffer2 : dspbuff3/Buffer  Orientation=left  N=8192  V=0  ic=0
  Complex to Real-Imag : ComplexToRealImag  Orientation=left  Output=Real
  Frame Conversion2 : FrameConversion  Orientation=left
  Frame Conversion3 : FrameConversion  Orientation=left  OutFrame=Sample-based
  IFFT : dspxfrm3/IFFT  Orientation=left  DialogController=dspDDGCreate  DialogControllerArgs=DataTag10  CompMethod=Table lookup  TableOpt=HYBRID  TableOptActive=Speed  BitRevOrder=off  cs_in=off  SkipNorm=on  InheritFFTLength=on  FFTLength=64  mode=Complex  outSamplingMode=Frame based  roundingMode=Floor  overflowMode=off
  Integer Delay : simulink/Discrete/Integer Delay  Orientation=left  vinit=0.0  samptime=-1  NumDelays=2048
  Magnitude-Angle to Complex : MagnitudeAngleToComplex  Orientation=left
  Unbuffer1 : dspbuff3/Unbuffer  Orientation=left  ic=0
  Unbuffer2 : dspbuff3/Unbuffer  Orientation=left  ic=0
  Out1 : Outport  Orientation=left  OutDataType=sfix(16)  OutScaling=2^0
  wires:
  Frame Conversion2/1 -> Unbuffer1/1
  Unbuffer1/1 -> Buffer2/1
  Buffer2/1 -> Frame Conversion3/1
  Magnitude-Angle to Complex/1 -> IFFT/1
  IFFT/1 -> Integer Delay/1
  Unbuffer2/1 -> Complex to Real-Imag/1
  Frame Conversion3/1 -> Magnitude-Angle to Complex/2
  Complex to Real-Imag/1 -> Out1/1
  In1/1 -> Frame Conversion2/1
  In2/1 -> Magnitude-Angle to Complex/1
  Integer Delay/1 -> Unbuffer2/1

== system dsss/Anti-interference/firstroad2/threshold ==
  In1 : Inport  OutDataType=sfix(16)  OutScaling=2^0
  Add1 : Sum  OutDataType=sfix(16)  OutScaling=2^-10
  Constant : Constant  Value=8192  OutDataType=sfix(16)  OutScaling=2^0
  Constant1 : Constant  Value=400  OutDataType=sfix(16)  OutScaling=2^0
  Display6 : Display
  Divide : Product  Inputs=*/  OutDataType=sfix(16)  OutScaling=2^-10
  Gain : Gain  Gain=0.3  ParameterDataType=sfix(16)  ParameterScaling=2^0  OutDataType=sfix(16)  OutScaling=2^0
  Matrix Sum : dspobslib/Matrix Sum  DialogController=dspDDGCreate  DialogControllerArgs=DataTag11  Dim=Columns  roundingMode=Floor  overflowMode=off
  Rate Transition1 : RateTransition  Deterministic=off  OutPortSampleTime=8192/5.1e6
  Rate Transition2 : RateTransition  Orientation=down  Deterministic=off  OutPortSampleTime=1/5.1e6
  Zero-Order Hold5 : ZeroOrderHold  SampleTime=1/5.1e6
  Out1 : Outport  OutDataType=sfix(16)  OutScaling=2^0
  wires:
  Matrix Sum/1 -> Divide/1
  Divide/1 -> Gain/1
  Gain/1 -> Rate Transition2/1
  Add1/1 -> Display6/1, Out1/1
  In1/1 -> Matrix Sum/1
  Constant1/1 -> Zero-Order Hold5/1
  Rate Transition1/1 -> Divide/2
  Constant/1 -> Rate Transition1/1
  Zero-Order Hold5/1 -> Add1/2
  Rate Transition2/1 -> Add1/1

== system dsss/Anti-interference/firstroad3/all ==
  In1 : Inport  OutDataType=sfix(16)  OutScaling=2^0
  Buffer1 : dspbuff3/Buffer  N=8192  V=0  ic=0
  FFT1 : dspxfrm3/FFT  DialogController=dspDDGCreate  DialogControllerArgs=DataTag12  CompMethod=Table lookup  TableOpt=HYBRID  TableOptActive=Speed  BitRevOrder=off  InheritFFTLength=on  FFTLength=64  SkipNorm=off  roundingMode=Floor  overflowMode=off
  Integer Delay : simulink/Discrete/Integer Delay  vinit=0.0  samptime=-1  NumDelays=6144
  Window Function : dspsigops/Window Function  DialogController=dspDDGCreate  DialogControllerArgs=DataTag13  winmode=Apply window to input  wintype=Chebyshev  sampmode=Continuous  samptime=1  N=64  Rs=80  beta=10  winsamp=Symmetric  UserWindow=hamming  OptParams=off  UserParams={'symmetric'}  dataType=double  isSigned=on  wordLen=16  udDataType=sfix(16)  fracBitsMode=Best precision  numFracBits=15  roundingMode=Floor  overflowMode=off  numSidelobes=4  sidelobeLevel=-30
  Out1 : Outport  OutDataType=sfix(16)  OutScaling=2^0
  wires:
  Window Function/1 -> FFT1/1
  In1/1 -> Buffer1/1
  FFT1/1 -> Out1/1
  Buffer1/1 -> Integer Delay/1
  Integer Delay/1 -> Window Function/1

== system dsss/Anti-interference/firstroad3/inteference_delieve ==
  In1 : Inport  OutDataType=sfix(16)  OutScaling=2^0
  In2 : Inport  Port=2  OutDataType=sfix(16)  OutScaling=2^0
  Buffer1 : dspbuff3/Buffer  N=8192  V=0  ic=0
  Frame Conversion : FrameConversion
  Frame Conversion1 : FrameConversion  Orientation=left  OutFrame=Sample-based
  Gain : Gain  Gain=0.1  ParameterDataType=sfix(16)  ParameterScaling=2^0  OutDataType=sfix(16)  OutScaling=2^0
  Subtract : Sum  Inputs=+-  OutDataType=sfix(16)  OutScaling=2^-10
  Switch : Switch
  Unbuffer : dspbuff3/Unbuffer  ic=0
  Out1 : Outport  Orientation=left  OutDataType=sfix(16)  OutScaling=2^0
  wires:
  Frame Conversion1/1 -> Out1/1
  In1/1 -> Frame Conversion/1
  Buffer1/1 -> Frame Conversion1/1
  Switch/1 -> Buffer1/1
  Gain/1 -> Switch/1
  Subtract/1 -> Switch/2
  In2/1 -> Gain/1, Subtract/2
  Frame Conversion/1 -> Unbuffer/1
  Unbuffer/1 -> Switch/3, Subtract/1

== system dsss/Anti-interference/firstroad3/inverse_convertion ==
  In1 : Inport  Orientation=left  OutDataType=sfix(16)  OutScaling=2^0
  In2 : Inport  Orientation=left  Port=2  OutDataType=sfix(16)  OutScaling=2^0
  Buffer2 : dspbuff3/Buffer  Orientation=left  N=8192  V=0  ic=0
  Complex to Real-Imag : ComplexToRealImag  Orientation=left  Output=Real
  Frame Conversion2 : FrameConversion  Orientation=left
  Frame Conversion3 : FrameConversion  Orientation=left  OutFrame=Sample-based
  IFFT : dspxfrm3/IFFT  Orientation=left  DialogController=dspDDGCreate  DialogControllerArgs=DataTag14  CompMethod=Table lookup  TableOpt=HYBRID  TableOptActive=Speed  BitRevOrder=off  cs_in=off  SkipNorm=on  InheritFFTLength=on  FFTLength=64  mode=Complex  outSamplingMode=Frame based  roundingMode=Floor  overflowMode=off
  Magnitude-Angle to Complex : MagnitudeAngleToComplex  Orientation=left
  Unbuffer1 : dspbuff3/Unbuffer  Orientation=left  ic=0
  Unbuffer2 : dspbuff3/Unbuffer  Orientation=left  ic=0
  Out1 : Outport  Orientation=left  OutDataType=sfix(16)  OutScaling=2^0
  wires:
  In2/1 -> Magnitude-Angle to Complex/1
  In1/1 -> Frame Conversion2/1
  Complex to Real-Imag/1 -> Out1/1
  Frame Conversion3/1 -> Magnitude-Angle to Complex/2
  Unbuffer2/1 -> Complex to Real-Imag/1
  IFFT/1 -> Unbuffer2/1
  Magnitude-Angle to Complex/1 -> IFFT/1
  Buffer2/1 -> Frame Conversion3/1
  Unbuffer1/1 -> Buffer2/1
  Frame Conversion2/1 -> Unbuffer1/1

== system dsss/Anti-interference/firstroad3/threshold ==
  In1 : Inport  OutDataType=sfix(16)  OutScaling=2^0
  Add1 : Sum  OutDataType=sfix(16)  OutScaling=2^-10
  Constant : Constant  Value=8192  OutDataType=sfix(16)  OutScaling=2^0
  Constant1 : Constant  Value=400  OutDataType=sfix(16)  OutScaling=2^0
  Display6 : Display
  Divide : Product  Inputs=*/  OutDataType=sfix(16)  OutScaling=2^-10
  Gain : Gain  Gain=0.3  ParameterDataType=sfix(16)  ParameterScaling=2^0  OutDataType=sfix(16)  OutScaling=2^0
  Matrix Sum : dspobslib/Matrix Sum  DialogController=dspDDGCreate  DialogControllerArgs=DataTag15  Dim=Columns  roundingMode=Floor  overflowMode=off
  Rate Transition1 : RateTransition  Deterministic=off  OutPortSampleTime=8192/5.1e6
  Rate Transition2 : RateTransition  Orientation=down  Deterministic=off  OutPortSampleTime=1/5.1e6
  Zero-Order Hold5 : ZeroOrderHold  SampleTime=1/5.1e6
  Out1 : Outport  OutDataType=sfix(16)  OutScaling=2^0
  wires:
  Rate Transition2/1 -> Add1/1
  Zero-Order Hold5/1 -> Add1/2
  Constant/1 -> Rate Transition1/1
  Rate Transition1/1 -> Divide/2
  Constant1/1 -> Zero-Order Hold5/1
  In1/1 -> Matrix Sum/1
  Add1/1 -> Out1/1, Display6/1
  Gain/1 -> Rate Transition2/1
  Divide/1 -> Gain/1
  Matrix Sum/1 -> Divide/1

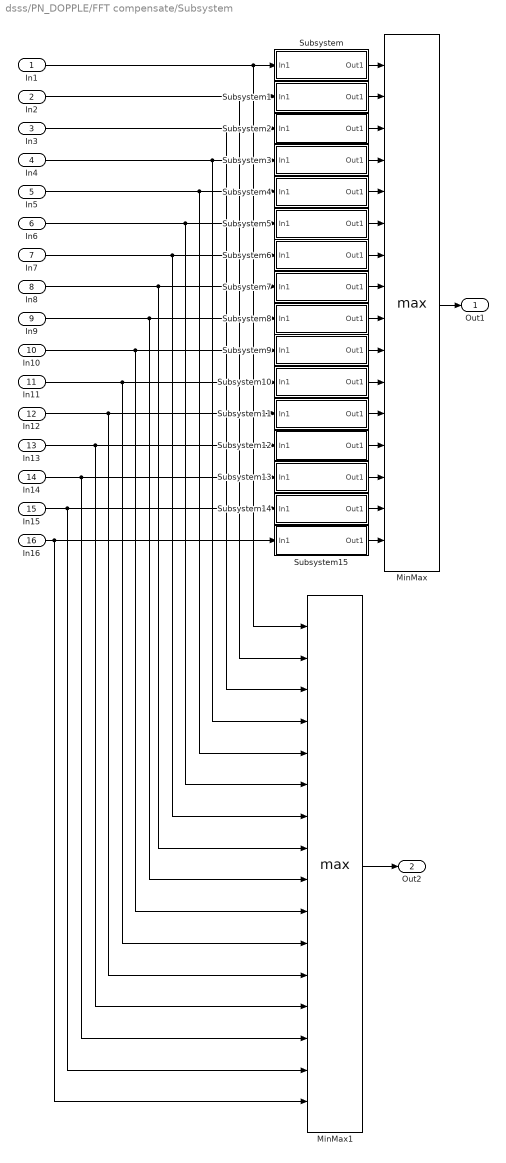
== system dsss/PN_DOPPLE/FFT compensate/Subsystem ==
  In1 : Inport  OutDataType=sfix(16)  OutScaling=2^0
  In2 : Inport  Port=2  OutDataType=sfix(16)  OutScaling=2^0
  In3 : Inport  Port=3  OutDataType=sfix(16)  OutScaling=2^0
  In4 : Inport  Port=4  OutDataType=sfix(16)  OutScaling=2^0
  In5 : Inport  Port=5  OutDataType=sfix(16)  OutScaling=2^0
  In6 : Inport  Port=6  OutDataType=sfix(16)  OutScaling=2^0
  In7 : Inport  Port=7  OutDataType=sfix(16)  OutScaling=2^0
  In8 : Inport  Port=8  OutDataType=sfix(16)  OutScaling=2^0
  In9 : Inport  Port=9  OutDataType=sfix(16)  OutScaling=2^0
  In10 : Inport  Port=10  OutDataType=sfix(16)  OutScaling=2^0
  In11 : Inport  Port=11  OutDataType=sfix(16)  OutScaling=2^0
  In12 : Inport  Port=12  OutDataType=sfix(16)  OutScaling=2^0
  In13 : Inport  Port=13  OutDataType=sfix(16)  OutScaling=2^0
  In14 : Inport  Port=14  OutDataType=sfix(16)  OutScaling=2^0
  In15 : Inport  Port=15  OutDataType=sfix(16)  OutScaling=2^0
  In16 : Inport  Port=16  OutDataType=sfix(16)  OutScaling=2^0
  MinMax : MinMax  Function=max  Inputs=16  OutDataType=sfix(16)  OutScaling=2^0
  MinMax1 : MinMax  Function=max  Inputs=16  OutDataType=sfix(16)  OutScaling=2^0
  Subsystem : Subsystem
  Subsystem1 : Subsystem
  Subsystem10 : Subsystem
  Subsystem11 : Subsystem
  Subsystem12 : Subsystem
  Subsystem13 : Subsystem
  Subsystem14 : Subsystem
  Subsystem15 : Subsystem
  Subsystem2 : Subsystem
  Subsystem3 : Subsystem
  Subsystem4 : Subsystem
  Subsystem5 : Subsystem
  Subsystem6 : Subsystem
  Subsystem7 : Subsystem
  Subsystem8 : Subsystem
  Subsystem9 : Subsystem
  Out1 : Outport  OutDataType=sfix(16)  OutScaling=2^0
  Out2 : Outport  Port=2  OutDataType=sfix(16)  OutScaling=2^0
  wires:
  In1/1 -> Subsystem/1(In1), MinMax1/1
  In2/1 -> Subsystem1/1(In1), MinMax1/2
  In3/1 -> Subsystem2/1(In1), MinMax1/3
  In4/1 -> Subsystem3/1(In1), MinMax1/4
  In5/1 -> Subsystem4/1(In1), MinMax1/5
  In6/1 -> Subsystem5/1(In1), MinMax1/6
  In7/1 -> Subsystem6/1(In1), MinMax1/7
  In8/1 -> Subsystem7/1(In1), MinMax1/8
  In9/1 -> Subsystem8/1(In1), MinMax1/9
  In10/1 -> Subsystem9/1(In1), MinMax1/10
  In11/1 -> Subsystem10/1(In1), MinMax1/11
  In12/1 -> Subsystem11/1(In1), MinMax1/12
  In13/1 -> Subsystem12/1(In1), MinMax1/13
  In14/1 -> Subsystem13/1(In1), MinMax1/14
  In15/1 -> Subsystem14/1(In1), MinMax1/15
  In16/1 -> Subsystem15/1(In1), MinMax1/16
  MinMax/1 -> Out1/1
  Subsystem/1(Out1) -> MinMax/1
  Subsystem1/1(Out1) -> MinMax/2
  Subsystem2/1(Out1) -> MinMax/3
  Subsystem3/1(Out1) -> MinMax/4
  Subsystem4/1(Out1) -> MinMax/5
  Subsystem5/1(Out1) -> MinMax/6
  Subsystem6/1(Out1) -> MinMax/7
  Subsystem7/1(Out1) -> MinMax/8
  Subsystem8/1(Out1) -> MinMax/9
  Subsystem9/1(Out1) -> MinMax/10
  Subsystem10/1(Out1) -> MinMax/11
  Subsystem11/1(Out1) -> MinMax/12
  Subsystem12/1(Out1) -> MinMax/13
  Subsystem13/1(Out1) -> MinMax/14
  Subsystem14/1(Out1) -> MinMax/15
  Subsystem15/1(Out1) -> MinMax/16
  MinMax1/1 -> Out2/1

== system dsss/PN_DOPPLE/Local PN/local PN sequence Include Track ==
  B : Inport  OutDataType=sfix(16)  OutScaling=2^0
  Enable : EnablePort  StatesWhenEnabling=reset
  Clock : Subsystem
  Local System : Subsystem
  Scope1 : Scope
      settings: YMin=0.95  YMax=1.05  SaveName=ScopeData10
  Scope2 : Scope
      settings: YMin=0.95  YMax=1.05  SaveName=ScopeData26
  Unipolar to Bipolar Converter : commutil2/Unipolar to Bipolar Converter  SystemSampleTime=-1  M=2  polarity=Positive  dataType=Inherit via internal rule
  "1 0 0 1 1 1 0 1 " : Outport  OutDataType=sfix(16)  OutScaling=2^0
  wires:
  Clock/1(Out1) -> Local System/1(In1), Scope1/1
  Local System/1("[1 0 0 1 1 1 0 1]") -> Unipolar to Bipolar Converter/1
  B/1 -> Clock/1(In2), Scope2/1
  Unipolar to Bipolar Converter/1 -> "1 0 0 1 1 1 0 1 "/1

== system dsss/PN_DOPPLE/Local PN/logic control ==
  In1 : Inport  OutDataType=sfix(16)  OutScaling=2^0
  Triggered Subsystem : Subsystem  TreatAsAtomicUnit=on
  Out2 : Outport  OutDataType=sfix(16)  OutScaling=2^0
  wires:
  Triggered Subsystem/1(Out2) -> Out2/1
  In1/1 -> Triggered Subsystem/Trigger

== system dsss/PN_DOPPLE/Local PN/threshold deside ==
  In1 : Inport  OutDataType=sfix(16)  OutScaling=2^0
  Enable : EnablePort
  Data Type Conversion : DataTypeConversion  OutDataTypeMode=double  OutDataType=sfix(16)  OutScaling=2^0  OutDataTypeStr=double
  Relational Operator : RelationalOperator  Operator=>  LogicOutDataTypeMode=boolean  OutDataTypeStr=boolean
  Scope : Scope
  Scope1 : Scope
      settings: SaveName=ScopeData28
  gate value : Constant  Value=60  OutDataType=sfix(16)  OutScaling=2^0
  Out2 : Outport  OutDataType=sfix(16)  OutScaling=2^0
  wires:
  In1/1 -> Relational Operator/1, Scope1/1
  gate value/1 -> Relational Operator/2
  Relational Operator/1 -> Scope/1, Data Type Conversion/1
  Data Type Conversion/1 -> Out2/1

== system dsss/PN_DOPPLE/Local PN/threshold deside stop and start ==
  In1 : Inport  OutDataType=sfix(16)  OutScaling=2^0
  In2 : Inport  Port=2  OutDataType=sfix(16)  OutScaling=2^0
  Constant : Constant  OutDataType=sfix(16)  OutScaling=2^0
  Logical Operator : Logic  Operator=XOR  AllPortsSameDT=off  OutDataTypeMode=boolean  OutDataTypeStr=boolean
  Logical Operator1 : Logic  Operator=OR  AllPortsSameDT=off  OutDataTypeMode=boolean  OutDataTypeStr=boolean
  Memory1 : Memory  InheritSampleTime=on
  Triggered Subsystem : Subsystem  TreatAsAtomicUnit=on
  Out1 : Outport  OutDataType=sfix(16)  OutScaling=2^0
  wires:
  Triggered Subsystem/1(Out1) -> Logical Operator/2
  Constant/1 -> Logical Operator/1
  Logical Operator/1 -> Memory1/1
  Memory1/1 -> Out1/1
  In1/1 -> Logical Operator1/2
  In2/1 -> Logical Operator1/1
  Logical Operator1/1 -> Triggered Subsystem/Trigger
